simulink model "ModelEnv_Test_Erreur_tracker"  (R2020b)
settings: Solver=VariableStepAuto  StartTime=0.0  StopTime=24  RelTol=1e-3
undefined symbols (not defined in the file): Atz, Bd, Bh, Tout, Tz_init
libraries: dspsrcs4 x2
settings Model: Creator=masdoua1  LastModifiedBy=masdoua1

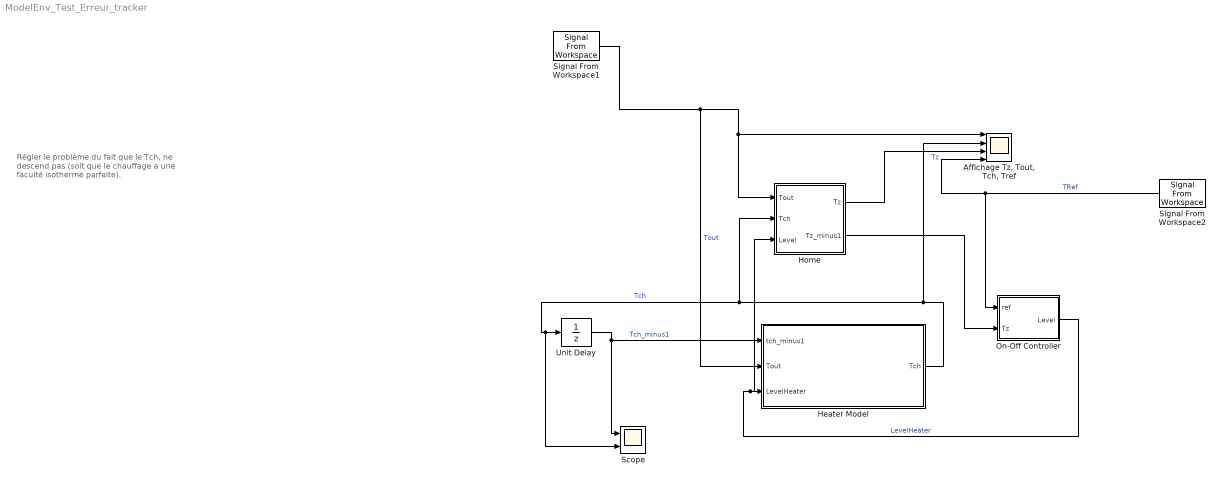
== system ModelEnv_Test_Erreur_tracker ==
  note: Régler le problème du fait que le Tch, ne descend pas (soit que le chauffage a une faculté isotherme parfaite).
  "Affichage Tz, Tout, Tch, Tref" : Scope  NumInputPorts=4
  Heater Model : Subsystem
  Home : Subsystem
  On-Off Controller : MATLAB Function  TreatAsAtomicUnit=on
  Scope : Scope  NumInputPorts=2
  Signal From Workspace1 : dspsrcs4/Signal From Workspace  X=Tout  Ts=1  nsamps=1  OutputAfterFinalValue=Setting to zero  ignoreOrWarnInputAndFrameLengths=off  OutputFrames=off
  Signal From Workspace2 : dspsrcs4/Signal From Workspace  X=Ref  Ts=1  nsamps=1  OutputAfterFinalValue=Setting to zero  ignoreOrWarnInputAndFrameLengths=off  OutputFrames=off
  Unit Delay : UnitDelay  InitialCondition=Tout(1)  SampleTime=-1  HasFrameUpgradeWarning=on
  wires:
  Unit Delay/1 -> Scope/1, Heater Model/1(tch_minus1)  "Tch_minus1"
  On-Off Controller/1(Level) -> Home/3(Level), Heater Model/3(LevelHeater)  "LevelHeater"
  Heater Model/1(Tch) -> "Affichage Tz, Tout, Tch, Tref"/2, Scope/2, Unit Delay/1, Home/2(Tch)  "Tch"
  Signal From Workspace1/1 -> Heater Model/2(Tout), Home/1(Tout), "Affichage Tz, Tout, Tch, Tref"/1  "Tout"
  Home/1(Tz) -> "Affichage Tz, Tout, Tch, Tref"/3  "Tz"
  Home/2(Tz_minus1) -> On-Off Controller/2(Tz)
  Signal From Workspace2/1 -> On-Off Controller/1(ref), "Affichage Tz, Tout, Tch, Tref"/4  "TRef"

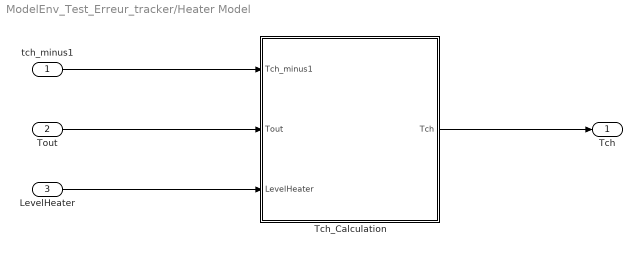
== system ModelEnv_Test_Erreur_tracker/Heater Model ==
  tch_minus1 : Inport
  Tout : Inport  Port=2
  LevelHeater : Inport  Port=3
  Tch_Calculation : MATLAB Function  TreatAsAtomicUnit=on
  Tch : Outport
  wires:
  Tout/1 -> Tch_Calculation/2(Tout)
  tch_minus1/1 -> Tch_Calculation/1(Tch_minus1)
  LevelHeater/1 -> Tch_Calculation/3(LevelHeater)
  Tch_Calculation/1(Tch) -> Tch/1

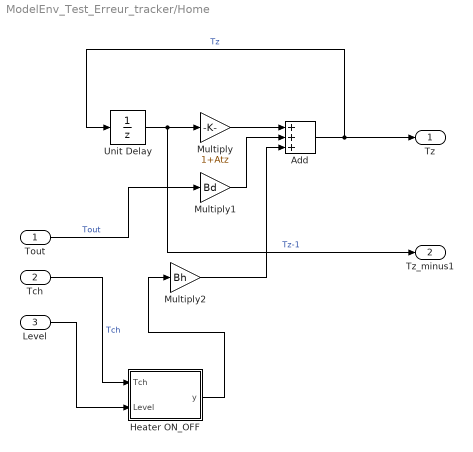
== system ModelEnv_Test_Erreur_tracker/Home ==
  Tout : Inport
  Tch : Inport  Port=2
  Level : Inport  Port=3
  Add : Sum  Inputs=+++
  Heater ON_OFF : MATLAB Function  TreatAsAtomicUnit=on
  Multiply : Gain  Gain=1+Atz
  Multiply1 : Gain  Gain=Bd
  Multiply2 : Gain  Gain=Bh
  Unit Delay : UnitDelay  InitialCondition=Tz_init  SampleTime=0.5  HasFrameUpgradeWarning=on
  Tz : Outport
  Tz_minus1 : Outport  Port=2
  wires:
  Multiply/1 -> Add/1
  Unit Delay/1 -> Tz_minus1/1, Multiply/1  "Tz-1"
  Tout/1 -> Multiply1/1  "Tout"
  Multiply1/1 -> Add/2
  Add/1 -> Unit Delay/1, Tz/1  "Tz"
  Multiply2/1 -> Add/3
  Level/1 -> Heater ON_OFF/2(Level)
  Tch/1 -> Heater ON_OFF/1(Tch)  "Tch"
  Heater ON_OFF/1(y) -> Multiply2/1

== matlab function ModelEnv_Test_Erreur_tracker/Heater Model/Tch_Calculation ==
  data: Tch_minus1 input; Tout input; LevelHeater input; Tch output
function Tch = fcn(Tch_minus1, Tout, LevelHeater)
    
    if Tout > Tch_minus1
        Tch_minus1 = Tout; 
    end
    
    Tch = Tch_minus1 + LevelHeater;

== matlab function ModelEnv_Test_Erreur_tracker/On-Off Controller ==
  data: ref input; Tz input; Level output
function Level= fcn(ref, Tz)

err = ref - Tz;

if err >= 7
    Level = 2;
elseif err >= 4
    Level = 1.14;
elseif err >= 1
    Level = 0.25;
else 
    Level = 0;
end

== matlab function ModelEnv_Test_Erreur_tracker/Home/Heater ON_OFF ==
  data: Tch input; Level input; y output
function y = fcn(Tch, Level)
y = Tch;
if Level ==0
        y = 0;
end
